simulink model "untitled1"  (R2016b)
settings: Solver=FixedStepAuto  StartTime=0.0  StopTime=0.3  FixedStep=0.00003  RelTol=1e-3
settings Model: Creator=Admin  LastModifiedBy=Admin

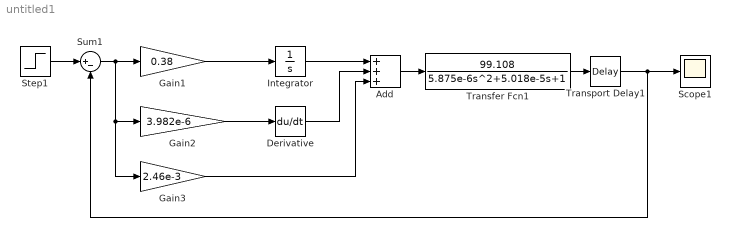
== system untitled1 ==
  Add : Sum  Inputs=+++
  Derivative : Derivative
  Gain1 : Gain  Gain=0.38
  Gain2 : Gain  Gain=3.982e-6
  Gain3 : Gain  Gain=2.46e-3
  Integrator : Integrator
  Scope1 : Scope
  Step1 : Step  Time=0  SampleTime=0
  Sum1 : Sum  Inputs=|+-
  Transfer Fcn1 : TransferFcn  Numerator=[99.108]  Denominator=[5.875e-6 5.018e-5 1]
  Transport Delay1 : TransportDelay  DelayTime=1.25e-4
  wires:
  Step1/1 -> Sum1/1
  Transfer Fcn1/1 -> Transport Delay1/1
  Sum1/1 -> Gain3/1, Gain2/1, Gain1/1
  Transport Delay1/1 -> Scope1/1, Sum1/2
  Gain1/1 -> Integrator/1
  Gain2/1 -> Derivative/1
  Add/1 -> Transfer Fcn1/1
  Derivative/1 -> Add/2
  Integrator/1 -> Add/1
  Gain3/1 -> Add/3
